simulink model "sampleModel1811"  (R2023a)
settings: Solver=VariableStepAuto  StartTime=0.0  StopTime=10.0  RelTol=1e-3
libraries: simulink x5, hdlsllib x4
settings Model: Creator=user1  LastModifiedBy=user1

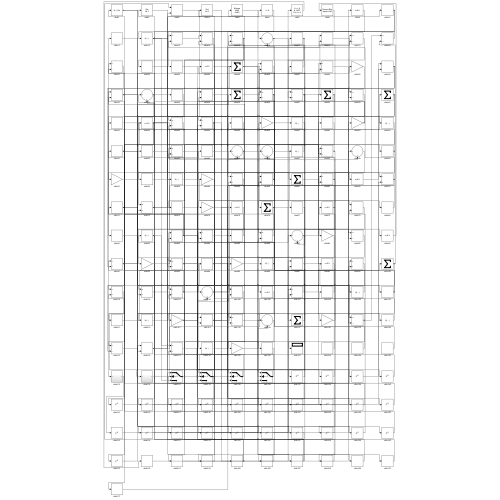
[thumbnail: Simulink's stored preview of the top-level diagram]
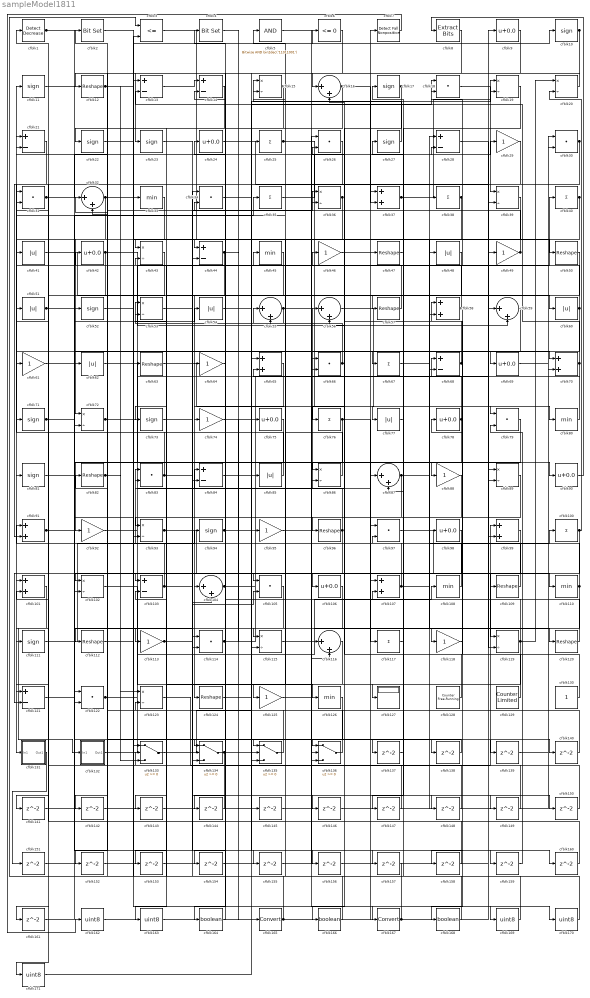
== system sampleModel1811 ==
  cfblk1 : simulink/Logic and Bit Operations/Detect Decrease  vinit=0.0  OutDataTypeStr=boolean
      settings: LibrarySourceBlock=|
      | hdlsllib/Logic and Bit
      | Operations/Detect
      | Decrease
  cfblk{10..11,17,22..23,27,52,71,73,81,94,111} (12 alike) : Signum
  cfblk{25,35,38,40,67,76,100,117} (8 alike) : Sum  Inputs=+
  cfblk{37,58,65,70,91,99,101,107} (8 alike) : Sum
  cfblk{15,19..20,36,39,43,53,72,86,89,93,102,115,119,123} (15 alike) : Product  Inputs=*/  RndMeth=Zero  SaturateOnIntegerOverflow=on
  cfblk{13..14,21,28,44,68,84,103,121} (9 alike) : Sum  Inputs=+-
  cfblk{16,32,55..56,59,87,104,116} (8 alike) : Sum  Inputs=|++
  cfblk{18,26,30..31,34,66,79,83,97,105,114,122} (12 alike) : DotProduct  OutDataTypeStr=Inherit: Inherit via internal rule
  cfblk{9,24,42,69,75,78,90,98,106} (9 alike) : Bias  Bias=0.0  SaturateOnIntegerOverflow=off
  cfblk{33,45,80,108,110,126} (6 alike) : MinMax
  cfblk{12,47,50,57,63,82,96,109,112,120,124} (11 alike) : Reshape
  cfblk{29,46,49,61,64,74,88,92,95,113,118,125} (12 alike) : Gain
  cfblk127 : Display
  cfblk128 : hdlsllib/Sources/Counter Free-Running  NumBits=16  tsamp=-1
  cfblk129 : hdlsllib/Sources/Counter Limited  uplimit=7  tsamp=-1
  cfblk130 : Constant  SampleTime=-1
  cfblk131 : Subsystem
      settings: LibrarySourceBlock=|
      | hdlsllib/Ports &
      | Subsystems/Subsystem
  cfblk132 : Subsystem
      settings: LibrarySourceBlock=|
      | hdlsllib/Ports &
      | Subsystems/Subsystem
  cfblk{133..136} (4 alike) : Switch  SaturateOnIntegerOverflow=off  InputSameDT=off
  cfblk{137..161} (25 alike) : Delay  SampleTime=1
  cfblk{162..163,169..171} (5 alike) : DataTypeConversion  OutDataTypeStr=uint8  SaturateOnIntegerOverflow=off  RndMeth=Floor
  cfblk164 : DataTypeConversion  OutDataTypeStr=boolean  SaturateOnIntegerOverflow=off  RndMeth=Floor
  cfblk165 : DataTypeConversion  SaturateOnIntegerOverflow=off  RndMeth=Floor
  cfblk166 : DataTypeConversion  OutDataTypeStr=boolean  SaturateOnIntegerOverflow=off  RndMeth=Floor
  cfblk167 : DataTypeConversion  SaturateOnIntegerOverflow=off  RndMeth=Floor
  cfblk168 : DataTypeConversion  OutDataTypeStr=boolean  SaturateOnIntegerOverflow=off  RndMeth=Floor
  cfblk2 : simulink/Logic and Bit Operations/Bit Set  iBit=0
      settings: LibrarySourceBlock=|
      | hdlsllib/Logic and Bit
      | Operations/Bit Set
  cfblk3 : RelationalOperator  Operator=<=  OutDataTypeStr=boolean  InputSameDT=off
  cfblk4 : simulink/Logic and Bit Operations/Bit Set  iBit=0
      settings: LibrarySourceBlock=|
      | hdlsllib/Logic and Bit
      | Operations/Bit Set
  cfblk{41,48,51,54,60,62,77,85} (8 alike) : Abs  SaturateOnIntegerOverflow=off
  cfblk5 : simulink/Logic and Bit Operations/Bitwise Operator  logicop=AND  UseBitMask=on  BitMask=bin2dec('11011001')  BitMaskRealWorld=Stored Integer
      settings: LibrarySourceBlock=|
      | hdlsllib/Logic and Bit
      | Operations/Bitwise
      | Operator
  cfblk6 : hdlsllib/Logic and Bit Operations/Compare To Zero  relop=<=  OutDataTypeStr=boolean
  cfblk7 : hdlsllib/Logic and Bit Operations/Detect Fall Nonpositive  vinit=0  OutDataTypeStr=boolean
  cfblk8 : simulink/Logic and Bit Operations/Extract Bits  bitsToExtract=Upper half  numBits=8  bitIdxRange=[0 7]  outScalingMode=Preserve fixed-point scaling
      settings: LibrarySourceBlock=|
      | hdlsllib/Logic and Bit
      | Operations/Extract Bits
  wires:
  cfblk102/1 -> cfblk126/1
  cfblk27/1 -> cfblk15/1
  cfblk19/1 -> cfblk44/1
  cfblk20/1 -> cfblk23/1
  cfblk65/1 -> cfblk124/1
  cfblk92/1 -> cfblk40/1
  cfblk14/1 -> cfblk72/1
  cfblk80/1 -> cfblk68/1
  cfblk57/1 -> cfblk45/1
  cfblk123/1 -> cfblk99/1
  cfblk3/1 -> cfblk65/1
  cfblk75/1 -> cfblk92/1
  cfblk97/1 -> cfblk110/1
  cfblk91/1 -> cfblk135/1, cfblk54/1
  cfblk39/1 -> cfblk68/2
  cfblk111/1 -> cfblk83/1
  cfblk114/1 -> cfblk49/1, cfblk75/1, cfblk66/2
  cfblk42/1 -> cfblk59/2, cfblk60/1, cfblk121/1, cfblk61/1, cfblk134/3
  cfblk48/1 -> cfblk136/2
  cfblk96/1 -> cfblk53/1, cfblk121/2
  cfblk47/1 -> cfblk127/1
  cfblk55/1 -> cfblk53/2, cfblk58/2
  cfblk85/1 -> cfblk11/1
  cfblk101/1 -> cfblk132/1(In1)
  cfblk38/1 -> cfblk115/1, cfblk103/1
  cfblk86/1 -> cfblk55/1
  cfblk8/1 -> cfblk16/1
  cfblk18/1 -> cfblk39/1
  cfblk6/1 -> cfblk104/1
  cfblk82/1 -> cfblk112/1, cfblk133/3
  cfblk25/1 -> cfblk79/1, cfblk90/1
  cfblk117/1 -> cfblk27/1
  cfblk133/1 -> cfblk85/1
  cfblk119/1 -> cfblk135/2, cfblk20/1, cfblk107/2
  cfblk36/1 -> cfblk131/1(In1), cfblk102/2
  cfblk1/1 -> cfblk52/1, cfblk89/2
  cfblk115/1 -> cfblk118/1
  cfblk103/1 -> cfblk44/2, cfblk31/2
  cfblk21/1 -> cfblk81/1
  cfblk100/1 -> cfblk20/2, cfblk153/1
  cfblk2/1 -> cfblk167/1
  cfblk104/1 -> cfblk56/1, cfblk18/2
  cfblk87/1 -> cfblk48/1, cfblk134/2
  cfblk128/1 -> cfblk84/1
  cfblk63/1 -> cfblk77/1
  cfblk69/1 -> cfblk30/1
  cfblk54/1 -> cfblk19/1
  cfblk59/1 -> cfblk101/1
  cfblk68/1 -> cfblk41/1, cfblk88/1
  cfblk60/1 -> cfblk18/1, cfblk158/1
  cfblk40/1 -> cfblk96/1, cfblk106/1
  cfblk122/1 -> cfblk37/1, cfblk94/1
  cfblk130/1 -> cfblk16/2
  cfblk56/1 -> cfblk80/1
  cfblk45/1 -> cfblk74/1
  cfblk136/1 -> cfblk32/1
  cfblk67/1 -> cfblk120/1
  cfblk106/1 -> cfblk113/1
  cfblk93/1 -> cfblk119/1, cfblk36/2
  cfblk44/1 -> cfblk73/1, cfblk144/1, cfblk145/1
  cfblk22/1 -> cfblk50/1
  cfblk4/1 -> cfblk165/1
  cfblk112/1 -> cfblk10/1
  cfblk90/1 -> cfblk8/1
  cfblk71/1 -> cfblk35/1, cfblk93/2
  cfblk79/1 -> cfblk87/2
  cfblk49/1 -> cfblk24/1, cfblk21/1
  cfblk37/1 -> cfblk19/2, cfblk57/1, cfblk147/1
  cfblk70/1 -> cfblk13/2, cfblk65/2
  cfblk52/1 -> cfblk70/1
  cfblk84/1 -> cfblk66/1
  cfblk94/1 -> cfblk149/1, cfblk150/1
  cfblk129/1 -> cfblk78/1
  cfblk30/1 -> cfblk111/1, cfblk102/1
  cfblk134/1 -> cfblk133/2, cfblk160/1
  cfblk62/1 -> cfblk86/1
  cfblk51/1 -> cfblk67/1, cfblk114/2
  cfblk9/1 -> cfblk12/1
  cfblk41/1 -> cfblk98/1
  cfblk12/1 -> cfblk63/1, cfblk123/1, cfblk6/1
  cfblk118/1 -> cfblk58/1
  cfblk78/1 -> cfblk46/1, cfblk135/3
  cfblk110/1 -> cfblk125/1, cfblk56/2, cfblk86/2
  cfblk13/1 -> cfblk14/1
  cfblk34/1 -> cfblk69/1
  cfblk108/1 -> cfblk15/2
  cfblk17/1 -> cfblk76/1, cfblk37/2
  cfblk132/1(Out1) -> cfblk108/1
  cfblk16/1 -> cfblk43/1, cfblk39/2
  cfblk58/1 -> cfblk42/1, cfblk168/1
  cfblk107/1 -> cfblk26/2, cfblk100/1
  cfblk31/1 -> cfblk105/1, cfblk29/1
  cfblk76/1 -> cfblk117/1, cfblk134/1
  cfblk26/1 -> cfblk84/2
  cfblk46/1 -> cfblk47/1
  cfblk120/1 -> cfblk71/1
  cfblk105/1 -> cfblk122/2
  cfblk10/1 -> cfblk62/1, cfblk115/2
  cfblk28/1 -> cfblk119/2
  cfblk24/1 -> cfblk89/1
  cfblk125/1 -> cfblk116/2
  cfblk83/1 -> cfblk51/1, cfblk21/2, cfblk139/1, cfblk140/1
  cfblk50/1 -> cfblk93/1
  cfblk124/1 -> cfblk25/1
  cfblk109/1 -> cfblk91/1
  cfblk135/1 -> cfblk43/2
  cfblk29/1 -> cfblk91/2
  cfblk66/1 -> cfblk31/1, cfblk36/1
  cfblk35/1 -> cfblk28/2
  cfblk11/1 -> cfblk109/1
  cfblk32/1 -> cfblk33/1, cfblk161/1
  cfblk113/1 -> cfblk105/2, cfblk157/1
  cfblk72/1 -> cfblk3/2, cfblk38/1
  cfblk15/1 -> cfblk64/1, cfblk22/1
  cfblk23/1 -> cfblk104/2
  cfblk77/1 -> cfblk137/1
  cfblk137/1 -> cfblk97/2
  cfblk53/1 -> cfblk138/1
  cfblk138/1 -> cfblk136/1
  cfblk139/1 -> cfblk70/2
  cfblk140/1 -> cfblk123/2
  cfblk43/1 -> cfblk141/1
  cfblk141/1 -> cfblk28/1
  cfblk98/1 -> cfblk142/1
  cfblk142/1 -> cfblk116/1
  cfblk88/1 -> cfblk143/1
  cfblk143/1 -> cfblk83/2
  cfblk144/1 -> cfblk32/2
  cfblk145/1 -> cfblk30/2
  cfblk73/1 -> cfblk146/1
  cfblk146/1 -> cfblk99/2
  cfblk147/1 -> cfblk101/2
  cfblk74/1 -> cfblk148/1
  cfblk148/1 -> cfblk34/2
  cfblk149/1 -> cfblk122/1
  cfblk150/1 -> cfblk14/2
  cfblk131/1(Out1) -> cfblk151/1
  cfblk151/1 -> cfblk26/1
  cfblk126/1 -> cfblk152/1
  cfblk152/1 -> cfblk59/1
  cfblk153/1 -> cfblk107/1
  cfblk89/1 -> cfblk154/1
  cfblk154/1 -> cfblk55/2
  cfblk81/1 -> cfblk155/1
  cfblk155/1 -> cfblk136/3
  cfblk121/1 -> cfblk156/1
  cfblk156/1 -> cfblk87/1
  cfblk157/1 -> cfblk3/1
  cfblk158/1 -> cfblk13/1
  cfblk61/1 -> cfblk159/1
  cfblk159/1 -> cfblk79/2
  cfblk160/1 -> cfblk1/1
  cfblk161/1 -> cfblk72/2
  cfblk7/1 -> cfblk162/1
  cfblk162/1 -> cfblk9/1
  cfblk116/1 -> cfblk163/1
  cfblk163/1 -> cfblk7/1
  cfblk64/1 -> cfblk164/1
  cfblk164/1 -> cfblk4/1
  cfblk165/1 -> cfblk114/1, cfblk34/1
  cfblk99/1 -> cfblk166/1
  cfblk166/1 -> cfblk2/1
  cfblk167/1 -> cfblk133/1, cfblk103/2, cfblk82/1
  cfblk168/1 -> cfblk5/1
  cfblk5/1 -> cfblk169/1
  cfblk169/1 -> cfblk17/1
  cfblk95/1 -> cfblk170/1
  cfblk170/1 -> cfblk97/1
  cfblk33/1 -> cfblk171/1
  cfblk171/1 -> cfblk95/1

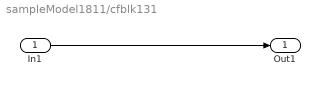
== system sampleModel1811/cfblk131 ==
  In1 : Inport
  Out1 : Outport
  wires:
  In1/1 -> Out1/1

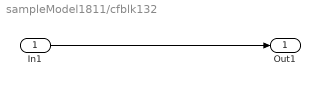
== system sampleModel1811/cfblk132 ==
  In1 : Inport
  Out1 : Outport
  wires:
  In1/1 -> Out1/1
